simulink model "Kpkikd2"  (R2023b)
settings: Solver=VariableStepAuto  StartTime=0.0  StopTime=10.0  RelTol=1e-3
settings Model: Creator=yasinsensoy  LastModifiedBy=yasinsensoy

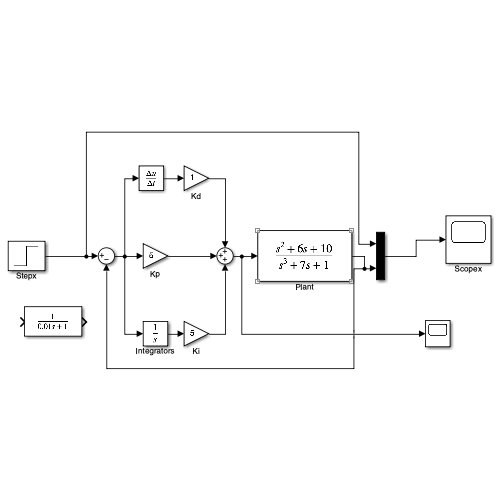
[thumbnail: Simulink's stored preview of the top-level diagram]
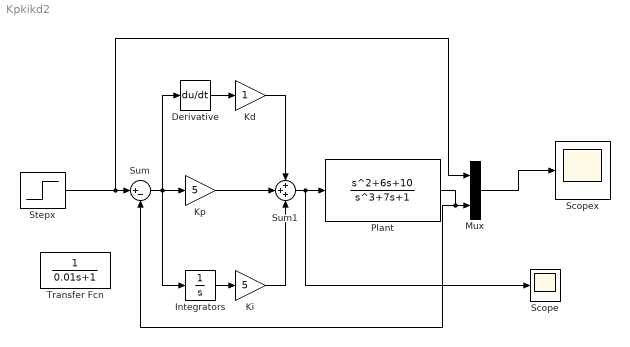
== system Kpkikd2 ==
  Derivative : Derivative
  Integrators : Integrator
  Kd : Gain
  Ki : Gain  Gain=5
  Kp : Gain  Gain=5
  Mux : Mux  Inputs=2
  Plant : TransferFcn  Numerator=[1 6 10]  Denominator=[1 0 7 1]
  Scope : Scope
  Scopex : Scope
  Stepx : Step  SampleTime=0
  Sum : Sum  Inputs=|+-
  Sum1 : Sum  Inputs=+++
  Transfer Fcn : TransferFcn  Denominator=[0.01 1]
  wires:
  Plant/1 -> Sum/2, Mux/2
  Stepx/1 -> Mux/1, Sum/1
  Mux/1 -> Scopex/1
  Integrators/1 -> Ki/1
  Sum1/1 -> Scope/1, Plant/1
  Sum/1 -> Derivative/1, Integrators/1, Kp/1
  Kd/1 -> Sum1/1
  Kp/1 -> Sum1/2
  Ki/1 -> Sum1/3
  Derivative/1 -> Kd/1
